simulink model "untitled"  (R2021b)
settings: Solver=VariableStepAuto  StartTime=0.0  StopTime=10.0  RelTol=1e-3
settings Model: Creator=Дмитрий  LastModifiedBy=Дмитрий

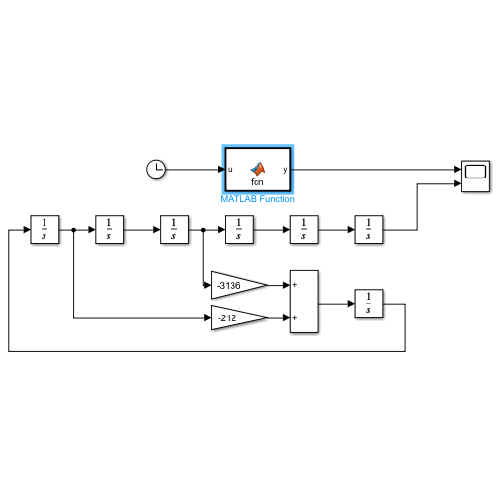
[thumbnail: Simulink's stored preview of the top-level diagram]
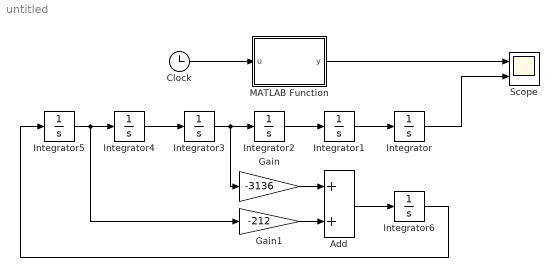
== system untitled ==
  Add : Sum
  Clock : Clock
  Gain : Gain  Gain=-3136
  Gain1 : Gain  Gain=-212
  Integrator{,1..6} (7 alike) : Integrator
  MATLAB Function : MATLAB Function  TreatAsAtomicUnit=on
  Scope : Scope  NumInputPorts=2
  wires:
  Clock/1 -> MATLAB Function/1(u)
  MATLAB Function/1(y) -> Scope/1
  Integrator/1 -> Scope/2
  Integrator1/1 -> Integrator/1
  Integrator2/1 -> Integrator1/1
  Integrator3/1 -> Gain/1, Integrator2/1
  Integrator4/1 -> Integrator3/1
  Integrator5/1 -> Gain1/1, Integrator4/1
  Gain/1 -> Add/1
  Gain1/1 -> Add/2
  Add/1 -> Integrator6/1
  Integrator6/1 -> Integrator5/1

== matlab function untitled/MATLAB Function ==
  data: u input; y output
function y = fcn(u)

y = cos(4*u)+cos(14*u)+3*u*u;
